simulink model "gyro_HS"  (R2018b)
settings: Solver=FixedStepAuto  StartTime=0.0  StopTime=10.0  RelTol=1e-3  EnableMultiTasking=on
libraries: legoev3lib x8, dspstat3 x1
settings Model: ExtModeTrigDuration=2  Creator=chpark  LastModifiedBy=chpark
settings SolverCC: PositivePriorityOrder=on
settings OptimizationCC: EnhancedBackFolding=on  PassReuseOutputArgsAs=Individual arguments  MaxStackSize=64  OptimizeBlockOrder=speed  DifferentSizesBufferReuse=on  OptimizationCustomize=off
settings DebuggingCC: ParameterTunabilityLossMsg=error
settings HardwareCC: ProdBitPerPointer=32  ProdBitPerSizeT=32  ProdBitPerPtrDiffT=32  ProdLargestAtomicInteger=Long  ProdWordSize=32  ProdHWDeviceType=ARM Compatible->ARM 9  UseEmbeddedCoderFeatures=off  UseSimulinkCoderFeatures=off
settings SFSimCC: MATLABDynamicMemAlloc=off
settings RTWCC: SystemTargetFile=ert.tlc  HardwareBoard=LEGO MINDSTORMS EV3  TLCOptions="-aInlineSetEventsForThisBaseRateFcn=TLC_FALSE -aSuppressMultiTaskScheduler=TLC_FALSE  -aRateBasedStepFcn=0"  TemplateMakefile=ert_default_tmf  GenerateReport=on  Toolchain=Sourcery G++ Lite v2009q3  IncludeHyperlinkInReport=on  LaunchReport=on  GenerateTraceInfo=on  GenerateTraceReport=on  GenerateTraceReportSl=on  GenerateTraceReportSf=on  GenerateTraceReportEml=on
settings CodeAppCC: ForceParamTrailComments=on  IgnoreCustomStorageClasses=off  OperatorAnnotations=on  SimulinkDataObjDesc=on  SFDataObjDesc=on  InsertBlockDesc=on
settings ERTTargetCC: SupportContinuousTime=on  SupportNonInlinedSFcns=on  SupportVariableSizeSignals=on

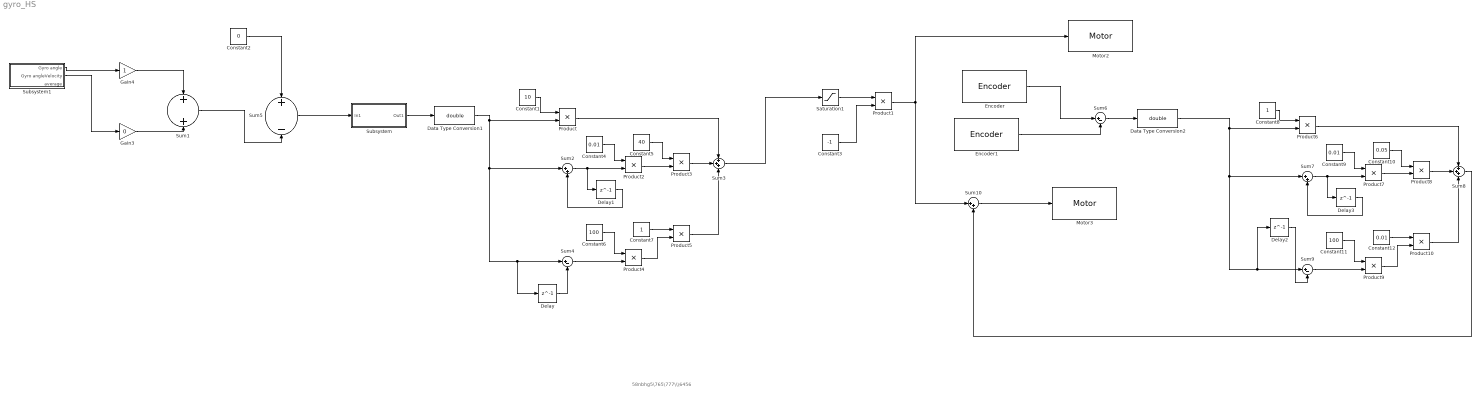
== system gyro_HS ==
  note: 58nbhg5\765\777\\\6456
  Constant1 : Constant  Value=10
  Constant10 : Constant  Value=0.05
  Constant11 : Constant  Value=100
  Constant12 : Constant  Value=0.01
  Constant2 : Constant  Value=0
  Constant3 : Constant  Value=-1
  Constant4 : Constant  Value=0.01
  Constant5 : Constant  Value=40
  Constant6 : Constant  Value=100
  Constant7 : Constant
  Constant8 : Constant
  Constant9 : Constant  Value=0.01
  Data Type Conversion1 : DataTypeConversion  OutDataTypeStr=double
  Data Type Conversion2 : DataTypeConversion  OutDataTypeStr=double
  Delay{,1..3} (4 alike) : Delay  DelayLength=1  InitialCondition=0
  Encoder : legoev3lib/Encoder  portNumber=A  opMode=Reset by external signal  sampleTime=0.01
      settings: SourceProductName=Simulink Support Package for LEGO MINDSTORMS EV3 Hardware  SourceProductBaseCode=LEGOEV3
  Encoder1 : legoev3lib/Encoder  portNumber=D  opMode=Reset by external signal  sampleTime=0.01
      settings: SourceProductName=Simulink Support Package for LEGO MINDSTORMS EV3 Hardware  SourceProductBaseCode=LEGOEV3
  Gain3 : Gain  Gain=0
  Gain4 : Gain
  Motor2 : legoev3lib/Motor  sportNumber=A  sstopAction=Brake
  Motor3 : legoev3lib/Motor  sportNumber=D  sstopAction=Brake
  Product{,1..10} (11 alike) : Product
  Saturation1 : Saturate  UpperLimit=100  LowerLimit=-100
  Subsystem : Subsystem
  Subsystem1 : Subsystem
  Sum1 : Sum
  Sum10 : Sum  Inputs=|++
  Sum2 : Sum  Inputs=|++
  Sum3 : Sum  Inputs=+++
  Sum4 : Sum  Inputs=|+-
  Sum5 : Sum  Inputs=+-
  Sum6 : Sum  Inputs=|+-
  Sum7 : Sum  Inputs=|++
  Sum8 : Sum  Inputs=+++
  Sum9 : Sum  Inputs=|+-
  wires:
  Constant6/1 -> Product4/1
  Sum2/1 -> Delay1/1, Product2/2
  Sum4/1 -> Product4/2
  Gain4/1 -> Sum1/1
  Constant8/1 -> Product6/1
  Subsystem/1(Out1) -> Data Type Conversion1/1
  Data Type Conversion1/1 -> Delay/1, Sum4/1, Sum2/1, Product/2
  Sum8/1 -> Sum10/2
  Gain3/1 -> Sum1/2
  Sum10/1 -> Motor3/1
  Delay/1 -> Sum4/2
  Constant11/1 -> Product9/1
  Subsystem1/1(Gyro angle) -> Gain4/1
  Delay3/1 -> Sum7/2
  Delay2/1 -> Sum9/2
  Constant4/1 -> Product2/1
  Constant9/1 -> Product7/1
  Data Type Conversion2/1 -> Delay2/1, Sum9/1, Sum7/1, Product6/2
  Product8/1 -> Sum8/2
  Sum1/1 -> Sum5/2
  Constant1/1 -> Product/1
  Delay1/1 -> Sum2/2
  Sum9/1 -> Product9/2
  Product6/1 -> Sum8/1
  Constant10/1 -> Product8/1
  Product7/1 -> Product8/2
  Product/1 -> Sum3/1
  Sum7/1 -> Delay3/1, Product7/2
  Constant12/1 -> Product10/1
  Constant7/1 -> Product5/1
  Product10/1 -> Sum8/3
  Sum6/1 -> Data Type Conversion2/1
  Product2/1 -> Product3/2
  Product1/1 -> Sum10/1, Motor2/1
  Constant3/1 -> Product1/2
  Subsystem1/2(Gyro angleVelocity) -> Gain3/1
  Constant2/1 -> Sum5/1
  Saturation1/1 -> Product1/1
  Sum3/1 -> Saturation1/1
  Product5/1 -> Sum3/3
  Product4/1 -> Product5/2
  Encoder/1 -> Sum6/1
  Product3/1 -> Sum3/2
  Constant5/1 -> Product3/1
  Sum5/1 -> Subsystem/1(In1)
  Encoder1/1 -> Sum6/2
  Product9/1 -> Product10/2

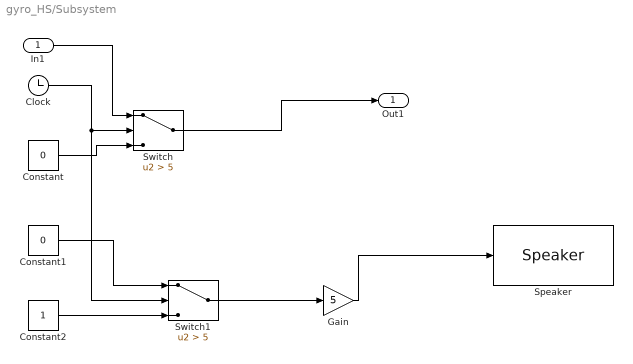
== system gyro_HS/Subsystem ==
  In1 : Inport
  Clock : Clock
  Constant : Constant  Value=0
  Constant1 : Constant  Value=0
  Constant2 : Constant
  Gain : Gain  Gain=5
  Speaker : legoev3lib/Speaker  sinputMode=Volume only  sspeakerFreq=100  sspeakerVolume=50  sspeakerDuration=100
      settings: SourceProductName=Simulink Support Package for LEGO MINDSTORMS EV3 Hardware  SourceProductBaseCode=LEGOEV3
  Switch : Switch  Criteria=u2 > Threshold  Threshold=5
  Switch1 : Switch  Criteria=u2 > Threshold  Threshold=5
  Out1 : Outport
  wires:
  Clock/1 -> Switch1/2, Switch/2
  In1/1 -> Switch/1
  Constant/1 -> Switch/3
  Constant1/1 -> Switch1/1
  Constant2/1 -> Switch1/3
  Gain/1 -> Speaker/1
  Switch1/1 -> Gain/1
  Switch/1 -> Out1/1

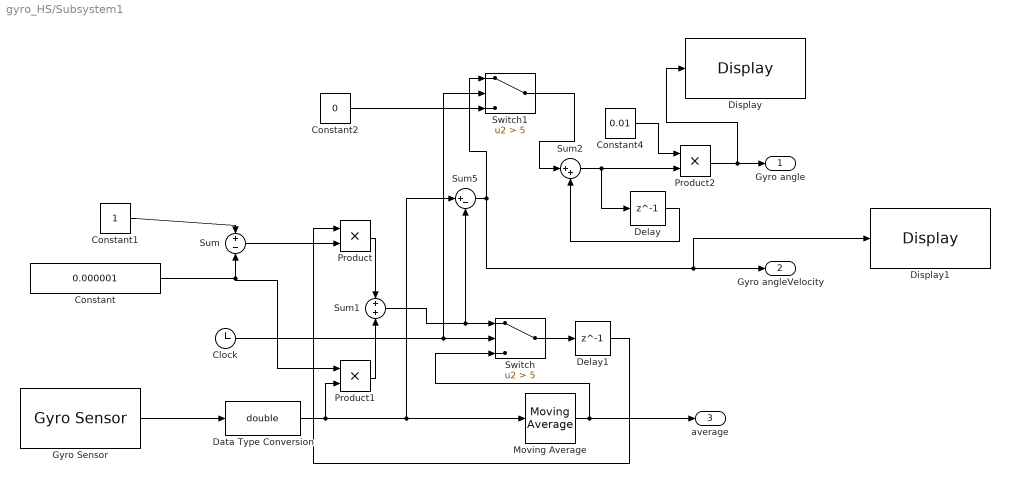
== system gyro_HS/Subsystem1 ==
  Clock : Clock
  Constant : Constant  Value=0.000001
  Constant1 : Constant
  Constant2 : Constant  Value=0
  Constant4 : Constant  Value=0.01
  Data Type Conversion : DataTypeConversion  OutDataTypeStr=double
  Delay : Delay  DelayLength=1  InitialCondition=0
  Delay1 : Delay  DelayLength=1  InitialCondition=0
  Display : legoev3lib/Display  slcdLine=3  slcdFormat=Decimal
      settings: SourceProductName=Simulink Support Package for LEGO MINDSTORMS EV3 Hardware  SourceProductBaseCode=LEGOEV3
  Display1 : legoev3lib/Display  slcdLine=5  slcdFormat=Decimal
      settings: SourceProductName=Simulink Support Package for LEGO MINDSTORMS EV3 Hardware  SourceProductBaseCode=LEGOEV3
  Gyro Sensor : legoev3lib/Gyro Sensor  portNumber=2  sampleTime=0.01
      settings: SourceProductName=Simulink Support Package for LEGO MINDSTORMS EV3 Hardware  SourceProductBaseCode=LEGOEV3
  Moving Average : dspstat3/Moving Average  Method=Sliding window  ForgettingFactorPort=off  SpecifyWindowLength=on  WindowLength=300  ForgettingFactor=0.9  SimulateUsing=Code generation
  Product : Product
  Product1 : Product
  Product2 : Product
  Sum : Sum  Inputs=+-
  Sum1 : Sum
  Sum2 : Sum  Inputs=|++
  Sum5 : Sum  Inputs=|+-
  Switch : Switch  Criteria=u2 > Threshold  Threshold=5
  Switch1 : Switch  Criteria=u2 > Threshold  Threshold=5
  Gyro angle : Outport
  Gyro angleVelocity : Outport  Port=2
  average : Outport  Port=3
  wires:
  Switch/1 -> Delay1/1
  Gyro Sensor/1 -> Data Type Conversion/1
  Moving Average/1 -> average/1, Switch/3
  Data Type Conversion/1 -> Product1/2, Moving Average/1, Sum5/1
  Sum5/1 -> Switch1/1, Display1/1, Gyro angleVelocity/1
  Clock/1 -> Switch1/2, Switch/2
  Constant1/1 -> Sum/1
  Constant/1 -> Product1/1, Sum/2
  Sum/1 -> Product/2
  Product/1 -> Sum1/1
  Product1/1 -> Sum1/2
  Sum1/1 -> Sum5/2, Switch/1
  Delay1/1 -> Product/1
  Constant4/1 -> Product2/1
  Delay/1 -> Sum2/2
  Product2/1 -> Display/1, Gyro angle/1
  Sum2/1 -> Delay/1, Product2/2
  Constant2/1 -> Switch1/3
  Switch1/1 -> Sum2/1
